simulink model "que3"  (R2023a)
settings: Solver=VariableStepAuto  StartTime=0.0  StopTime=50  RelTol=1e-3
settings Model: Creator=Administrator  LastModifiedBy=Administrator
settings SolverCC: AlgebraicLoopSolver=TrustRegion
settings DebuggingCC: ArithmeticOperatorsInVariantConditions=warning
settings SFSimCC: CustomCodeUndefinedFunction=UseInterfaceOnly

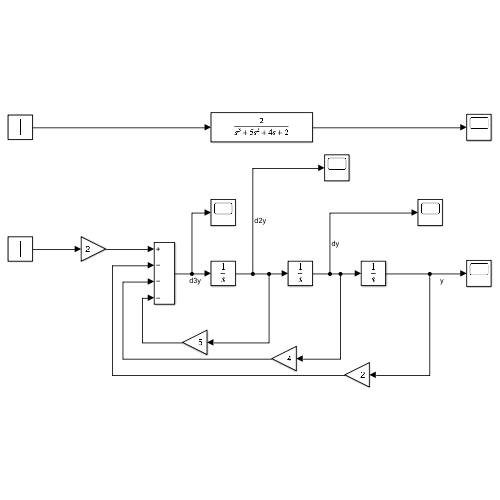
[thumbnail: Simulink's stored preview of the top-level diagram]
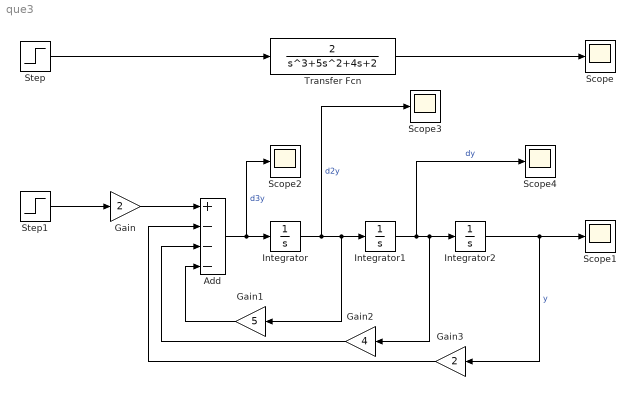
== system que3 ==
  Add : Sum  Inputs=+---
  Gain : Gain  Gain=2
  Gain1 : Gain  Gain=5
  Gain2 : Gain  Gain=4
  Gain3 : Gain  Gain=2
  Integrator : Integrator
  Integrator1 : Integrator
  Integrator2 : Integrator
  Scope{,1..4} (5 alike) : Scope
  Step : Step  SampleTime=0
  Step1 : Step  SampleTime=0
  Transfer Fcn : TransferFcn  Numerator=[2]  Denominator=[1 5 4 2]
  wires:
  Transfer Fcn/1 -> Scope/1
  Step/1 -> Transfer Fcn/1
  Add/1 -> Scope2/1, Integrator/1  "d3y"
  Integrator/1 -> Integrator1/1, Gain1/1, Scope3/1  "d2y"
  Integrator1/1 -> Scope4/1, Integrator2/1, Gain2/1  "dy"
  Gain1/1 -> Add/4
  Gain2/1 -> Add/3
  Integrator2/1 -> Scope1/1, Gain3/1  "y"
  Gain3/1 -> Add/2
  Gain/1 -> Add/1
  Step1/1 -> Gain/1
